simulink model "lab1_state_feedback_windup"  (R2024b)
settings: Solver=ode45  StartTime=0.0  StopTime=sIn.simulation_time
undefined symbols (not defined in the file or in its folder): degs2rpm, drv, feedback, filt, gbox, mld, mot, rads2rpm, rpm2rads, sens
libraries: simulink_extras x2, simulink x1
settings Model: Creator=bmm1  LastModifiedBy=pries
settings DataIOCC: ReturnWorkspaceOutputs=off
settings RTWCC: GPUComputeCapability=3.5

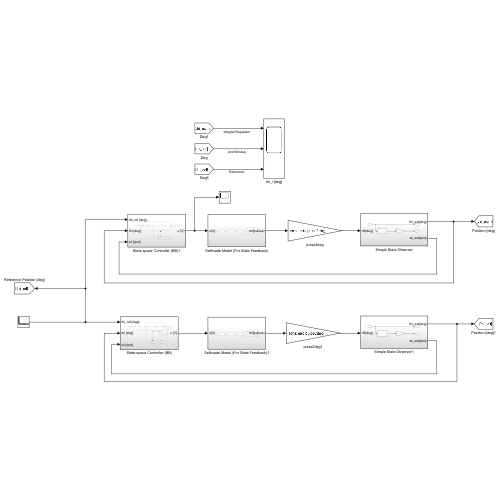
[thumbnail: Simulink's stored preview of the top-level diagram]
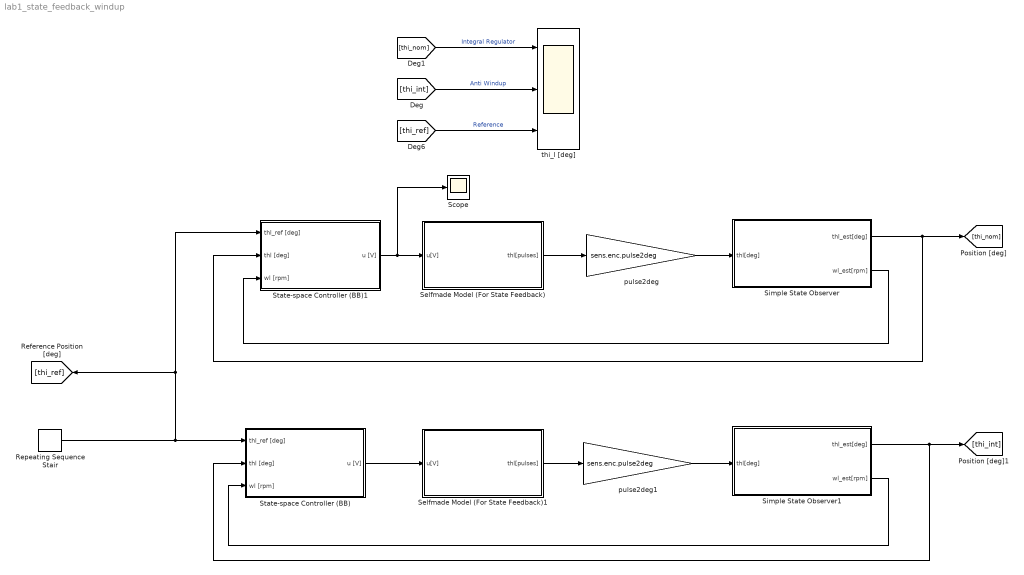
== system lab1_state_feedback_windup ==
  Repeating Sequence Stair : simulink/Sources/Repeating Sequence Stair  OutValues=sIn.position  tsamp=sIn.sample_time  OutMin=[]  OutMax=[]  OutDataTypeStr=double  OutputDataTypeScalingMode=double  OutDataType=fixdt(0,8)  ConRadixGroup=Best Precision: Vector-wise  OutScaling=2^-12
  Scope : Scope
  Selfmade Model (For State Feedback) : Subsystem
  Selfmade Model (For State Feedback)1 : Subsystem
  Simple State Observer : Subsystem
  Simple State Observer1 : Subsystem
  State-space Controller (BB) : Subsystem
  State-space Controller (BB)1 : Subsystem
  pulse2deg : Gain  Gain=sens.enc.pulse2deg
  pulse2deg1 : Gain  Gain=sens.enc.pulse2deg
  thi_l [deg] : Scope  NumInputPorts=3
  wires:
  Selfmade Model (For State Feedback)/1(thl[pulses]) -> pulse2deg/1
  Simple State Observer/1(thl_est[deg]) -> State-space Controller (BB)1/2(thl [deg]), [thi_nom]
  Simple State Observer/2(wl_est[rpm]) -> State-space Controller (BB)1/3(wl [rpm])
  State-space Controller (BB)1/1(u [V]) -> Scope/1, Selfmade Model (For State Feedback)/1(u[V])
  Repeating Sequence Stair/1 -> State-space Controller (BB)1/1(thl_ref [deg]), [thi_ref], State-space Controller (BB)/1(thl_ref [deg])
  State-space Controller (BB)/1(u [V]) -> Selfmade Model (For State Feedback)1/1(u[V])
  Selfmade Model (For State Feedback)1/1(thl[pulses]) -> pulse2deg1/1
  Simple State Observer1/1(thl_est[deg]) -> [thi_int], State-space Controller (BB)/2(thl [deg])
  Simple State Observer1/2(wl_est[rpm]) -> State-space Controller (BB)/3(wl [rpm])
  [thi_int] -> thi_l [deg]/2  "Anti Windup"
  [thi_nom] -> thi_l [deg]/1  "Integral Regulator"
  [thi_ref] -> thi_l [deg]/3  "Reference"
  pulse2deg1/1 -> Simple State Observer1/1(thl[deg])
  pulse2deg/1 -> Simple State Observer/1(thl[deg])

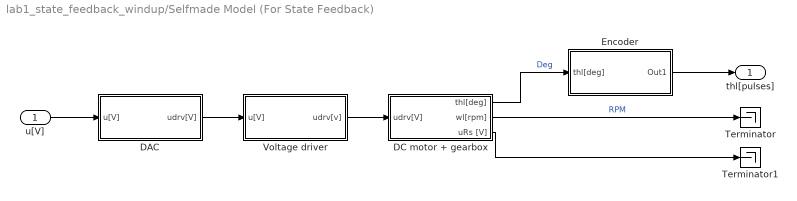
== system lab1_state_feedback_windup/Selfmade Model (For State Feedback) ==
  u[V] : Inport
  DAC : Subsystem
  DC motor + gearbox : Subsystem
  Encoder : Subsystem
  Terminator : Terminator
  Terminator1 : Terminator
  Voltage driver : Subsystem
  thl[pulses] : Outport
  wires:
  DC motor + gearbox/1(thl[deg]) -> Encoder/1(thl[deg])  "Deg"
  u[V]/1 -> DAC/1(u[V])
  DC motor + gearbox/2(wl[rpm]) -> Terminator/1  "RPM"
  DAC/1(udrv[V]) -> Voltage driver/1(u[V])
  Voltage driver/1(udrv[v]) -> DC motor + gearbox/1(udrv[V])
  Encoder/1(Out1) -> thl[pulses]/1
  DC motor + gearbox/3(uRs [V]) -> Terminator1/1

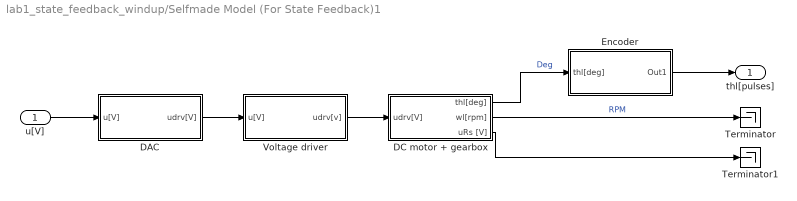
== system lab1_state_feedback_windup/Selfmade Model (For State Feedback)1 ==
  u[V] : Inport
  DAC : Subsystem
  DC motor + gearbox : Subsystem
  Encoder : Subsystem
  Terminator : Terminator
  Terminator1 : Terminator
  Voltage driver : Subsystem
  thl[pulses] : Outport
  wires:
  DC motor + gearbox/1(thl[deg]) -> Encoder/1(thl[deg])  "Deg"
  u[V]/1 -> DAC/1(u[V])
  DC motor + gearbox/2(wl[rpm]) -> Terminator/1  "RPM"
  DAC/1(udrv[V]) -> Voltage driver/1(u[V])
  Voltage driver/1(udrv[v]) -> DC motor + gearbox/1(udrv[V])
  Encoder/1(Out1) -> thl[pulses]/1
  DC motor + gearbox/3(uRs [V]) -> Terminator1/1

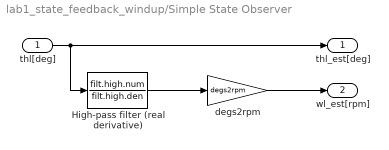
== system lab1_state_feedback_windup/Simple State Observer ==
  thl[deg] : Inport
  High-pass filter (real derivative) : TransferFcn  Numerator=filt.high.num  Denominator=filt.high.den
  degs2rpm : Gain  Gain=degs2rpm
  thl_est[deg] : Outport
  wl_est[rpm] : Outport  Port=2
  wires:
  thl[deg]/1 -> High-pass filter (real derivative)/1, thl_est[deg]/1
  High-pass filter (real derivative)/1 -> degs2rpm/1
  degs2rpm/1 -> wl_est[rpm]/1

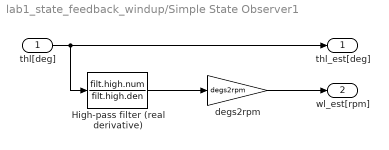
== system lab1_state_feedback_windup/Simple State Observer1 ==
  thl[deg] : Inport
  High-pass filter (real derivative) : TransferFcn  Numerator=filt.high.num  Denominator=filt.high.den
  degs2rpm : Gain  Gain=degs2rpm
  thl_est[deg] : Outport
  wl_est[rpm] : Outport  Port=2
  wires:
  thl[deg]/1 -> High-pass filter (real derivative)/1, thl_est[deg]/1
  High-pass filter (real derivative)/1 -> degs2rpm/1
  degs2rpm/1 -> wl_est[rpm]/1

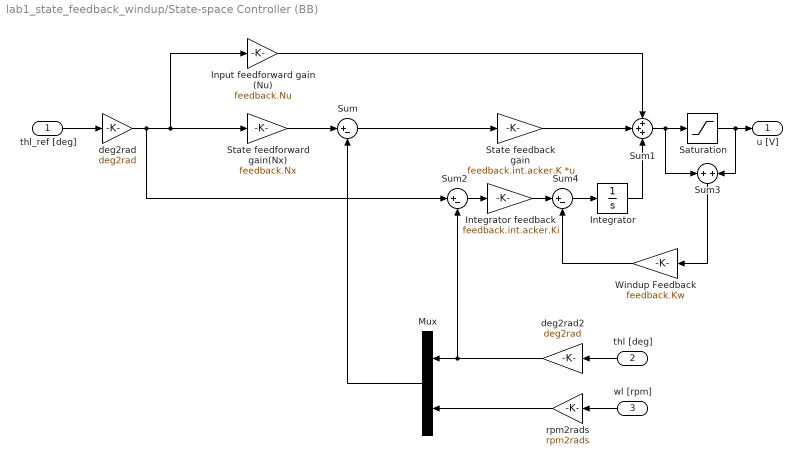
== system lab1_state_feedback_windup/State-space Controller (BB) ==
  thl_ref [deg] : Inport
  thl [deg] : Inport  Port=2
  wl [rpm] : Inport  Port=3
  Input feedforward gain (Nu) : Gain  Gain=feedback.Nu
  Integrator : Integrator
  Integrator feedback : Gain  Gain=feedback.int.acker.Ki
  Mux : Mux  Inputs=2
  Saturation : Saturate  UpperLimit=10  LowerLimit=-10
  State feedback gain : Gain  Gain=feedback.int.acker.K  Multiplication=Matrix(K*u)
  State feedforward gain(Nx) : Gain  Gain=feedback.Nx
  Sum : Sum  Inputs=|+-
  Sum1 : Sum  Inputs=+++
  Sum2 : Sum  Inputs=|+-
  Sum3 : Sum  Inputs=+|+
  Sum4 : Sum  Inputs=|+-
  Windup Feedback : Gain  Gain=feedback.Kw
  deg2rad : Gain  Gain=deg2rad
  deg2rad2 : Gain  Gain=deg2rad
  rpm2rads : Gain  Gain=rpm2rads
  u [V] : Outport
  wires:
  thl_ref [deg]/1 -> deg2rad/1
  deg2rad/1 -> Sum2/1, Input feedforward gain (Nu)/1, State feedforward gain(Nx)/1
  State feedforward gain(Nx)/1 -> Sum/1
  Sum/1 -> State feedback gain/1
  State feedback gain/1 -> Sum1/2
  Input feedforward gain (Nu)/1 -> Sum1/1
  Sum1/1 -> Sum3/1, Saturation/1
  Saturation/1 -> Sum3/2, u [V]/1
  thl [deg]/1 -> deg2rad2/1
  wl [rpm]/1 -> rpm2rads/1
  deg2rad2/1 -> Mux/1, Sum2/2
  rpm2rads/1 -> Mux/2
  Mux/1 -> Sum/2
  Sum2/1 -> Integrator feedback/1
  Integrator/1 -> Sum1/3
  Sum3/1 -> Windup Feedback/1
  Integrator feedback/1 -> Sum4/1
  Sum4/1 -> Integrator/1
  Windup Feedback/1 -> Sum4/2

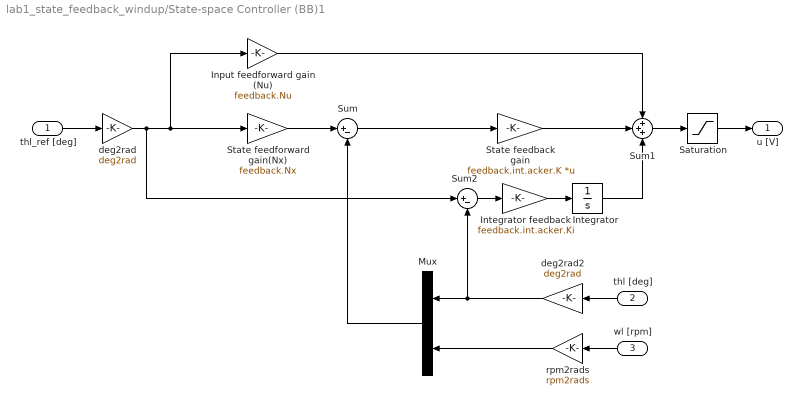
== system lab1_state_feedback_windup/State-space Controller (BB)1 ==
  thl_ref [deg] : Inport
  thl [deg] : Inport  Port=2
  wl [rpm] : Inport  Port=3
  Input feedforward gain (Nu) : Gain  Gain=feedback.Nu
  Integrator : Integrator
  Integrator feedback : Gain  Gain=feedback.int.acker.Ki
  Mux : Mux  Inputs=2
  Saturation : Saturate  UpperLimit=10  LowerLimit=-10
  State feedback gain : Gain  Gain=feedback.int.acker.K  Multiplication=Matrix(K*u)
  State feedforward gain(Nx) : Gain  Gain=feedback.Nx
  Sum : Sum  Inputs=|+-
  Sum1 : Sum  Inputs=+++
  Sum2 : Sum  Inputs=|+-
  deg2rad : Gain  Gain=deg2rad
  deg2rad2 : Gain  Gain=deg2rad
  rpm2rads : Gain  Gain=rpm2rads
  u [V] : Outport
  wires:
  thl_ref [deg]/1 -> deg2rad/1
  deg2rad/1 -> Sum2/1, Input feedforward gain (Nu)/1, State feedforward gain(Nx)/1
  State feedforward gain(Nx)/1 -> Sum/1
  Sum/1 -> State feedback gain/1
  State feedback gain/1 -> Sum1/2
  Input feedforward gain (Nu)/1 -> Sum1/1
  Sum1/1 -> Saturation/1
  Saturation/1 -> u [V]/1
  thl [deg]/1 -> deg2rad2/1
  wl [rpm]/1 -> rpm2rads/1
  deg2rad2/1 -> Sum2/2, Mux/1
  rpm2rads/1 -> Mux/2
  Mux/1 -> Sum/2
  Integrator feedback/1 -> Integrator/1
  Sum2/1 -> Integrator feedback/1
  Integrator/1 -> Sum1/3

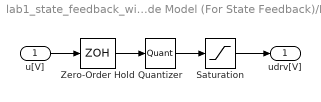
== system lab1_state_feedback_windup/Selfmade Model (For State Feedback)/DAC ==
  u[V] : Inport
  Quantizer : Quantizer  QuantizationInterval=daq.dac.q
  Saturation : Saturate  UpperLimit=10  LowerLimit=-10
  Zero-Order Hold : ZeroOrderHold  SampleTime=1e-3
  udrv[V] : Outport
  wires:
  Zero-Order Hold/1 -> Quantizer/1
  u[V]/1 -> Zero-Order Hold/1
  Quantizer/1 -> Saturation/1
  Saturation/1 -> udrv[V]/1

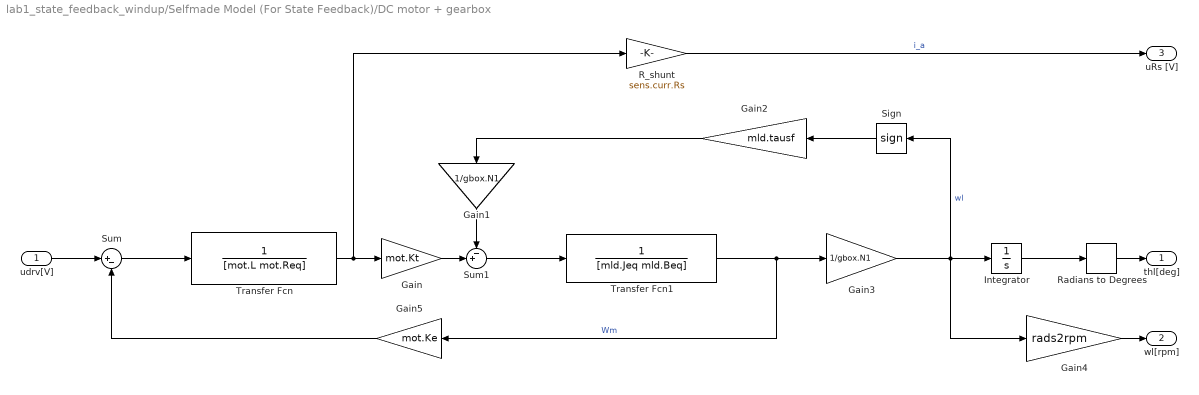
== system lab1_state_feedback_windup/Selfmade Model (For State Feedback)/DC motor + gearbox ==
  udrv[V] : Inport
  Gain : Gain  Gain=mot.Kt
  Gain1 : Gain  Gain=1/gbox.N1
  Gain2 : Gain  Gain=mld.tausf
  Gain3 : Gain  Gain=1/gbox.N1
  Gain4 : Gain  Gain=rads2rpm
  Gain5 : Gain  Gain=mot.Ke
  Integrator : Integrator
  R_shunt : Gain  Gain=sens.curr.Rs
  Radians to Degrees : simulink_extras/Transformations/Radians to Degrees
  Sign : Signum  ZeroCross=off
  Sum : Sum  Inputs=|+-
  Sum1 : Sum  Inputs=-+|
  Transfer Fcn : TransferFcn  Denominator=[mot.L mot.Req]
  Transfer Fcn1 : TransferFcn  Denominator=[mld.Jeq mld.Beq]
  thl[deg] : Outport
  wl[rpm] : Outport  Port=2
  uRs [V] : Outport  Port=3
  wires:
  udrv[V]/1 -> Sum/1
  Sum/1 -> Transfer Fcn/1
  Transfer Fcn/1 -> R_shunt/1, Gain/1
  Gain1/1 -> Sum1/1
  Gain2/1 -> Gain1/1
  Sign/1 -> Gain2/1
  Transfer Fcn1/1 -> Gain5/1, Gain3/1  "Wm"
  Gain3/1 -> Gain4/1, Sign/1, Integrator/1  "wl"
  Integrator/1 -> Radians to Degrees/1
  Radians to Degrees/1 -> thl[deg]/1
  Gain4/1 -> wl[rpm]/1
  Sum1/1 -> Transfer Fcn1/1
  Gain/1 -> Sum1/2
  Gain5/1 -> Sum/2
  R_shunt/1 -> uRs [V]/1  "i_a"

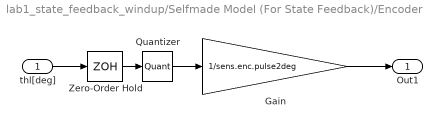
== system lab1_state_feedback_windup/Selfmade Model (For State Feedback)/Encoder ==
  thl[deg] : Inport
  Gain : Gain  Gain=1/sens.enc.pulse2deg
  Quantizer : Quantizer  QuantizationInterval=sens.enc.pulse2deg
  Zero-Order Hold : ZeroOrderHold  SampleTime=1e-3
  Out1 : Outport
  wires:
  thl[deg]/1 -> Zero-Order Hold/1
  Gain/1 -> Out1/1
  Quantizer/1 -> Gain/1
  Zero-Order Hold/1 -> Quantizer/1

== system lab1_state_feedback_windup/Selfmade Model (For State Feedback)/Voltage driver ==
  u[V] : Inport
  Saturation : Saturate  UpperLimit=12  LowerLimit=-12
  Transfer Fcn : TransferFcn  Numerator=[drv.dcgain]  Denominator=[drv.Tc 1]
  udrv[v] : Outport
  wires:
  u[V]/1 -> Transfer Fcn/1
  Transfer Fcn/1 -> Saturation/1
  Saturation/1 -> udrv[v]/1

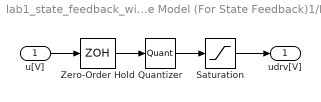
== system lab1_state_feedback_windup/Selfmade Model (For State Feedback)1/DAC ==
  u[V] : Inport
  Quantizer : Quantizer  QuantizationInterval=daq.dac.q
  Saturation : Saturate  UpperLimit=10  LowerLimit=-10
  Zero-Order Hold : ZeroOrderHold  SampleTime=1e-3
  udrv[V] : Outport
  wires:
  Zero-Order Hold/1 -> Quantizer/1
  u[V]/1 -> Zero-Order Hold/1
  Quantizer/1 -> Saturation/1
  Saturation/1 -> udrv[V]/1

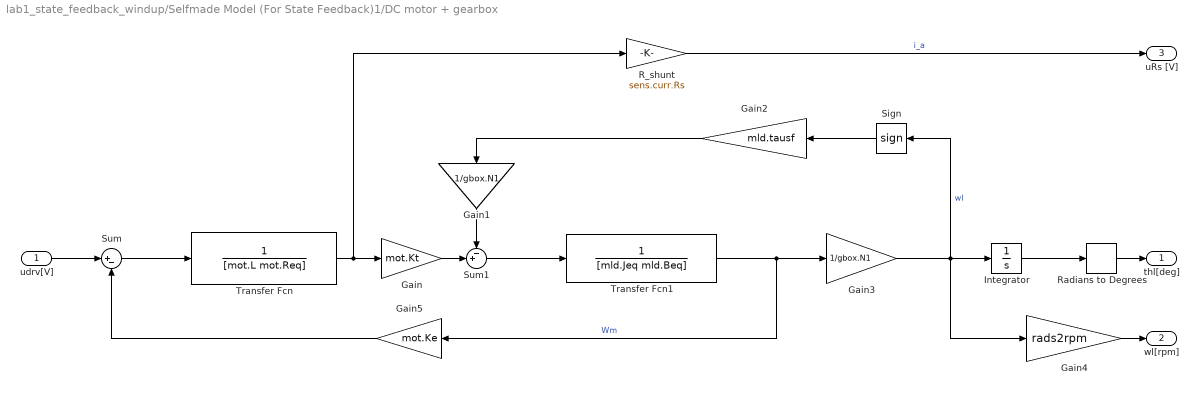
== system lab1_state_feedback_windup/Selfmade Model (For State Feedback)1/DC motor + gearbox ==
  udrv[V] : Inport
  Gain : Gain  Gain=mot.Kt
  Gain1 : Gain  Gain=1/gbox.N1
  Gain2 : Gain  Gain=mld.tausf
  Gain3 : Gain  Gain=1/gbox.N1
  Gain4 : Gain  Gain=rads2rpm
  Gain5 : Gain  Gain=mot.Ke
  Integrator : Integrator
  R_shunt : Gain  Gain=sens.curr.Rs
  Radians to Degrees : simulink_extras/Transformations/Radians to Degrees
  Sign : Signum  ZeroCross=off
  Sum : Sum  Inputs=|+-
  Sum1 : Sum  Inputs=-+|
  Transfer Fcn : TransferFcn  Denominator=[mot.L mot.Req]
  Transfer Fcn1 : TransferFcn  Denominator=[mld.Jeq mld.Beq]
  thl[deg] : Outport
  wl[rpm] : Outport  Port=2
  uRs [V] : Outport  Port=3
  wires:
  udrv[V]/1 -> Sum/1
  Sum/1 -> Transfer Fcn/1
  Transfer Fcn/1 -> R_shunt/1, Gain/1
  Gain1/1 -> Sum1/1
  Gain2/1 -> Gain1/1
  Sign/1 -> Gain2/1
  Transfer Fcn1/1 -> Gain5/1, Gain3/1  "Wm"
  Gain3/1 -> Gain4/1, Sign/1, Integrator/1  "wl"
  Integrator/1 -> Radians to Degrees/1
  Radians to Degrees/1 -> thl[deg]/1
  Gain4/1 -> wl[rpm]/1
  Sum1/1 -> Transfer Fcn1/1
  Gain/1 -> Sum1/2
  Gain5/1 -> Sum/2
  R_shunt/1 -> uRs [V]/1  "i_a"

== system lab1_state_feedback_windup/Selfmade Model (For State Feedback)1/Encoder ==
  thl[deg] : Inport
  Gain : Gain  Gain=1/sens.enc.pulse2deg
  Quantizer : Quantizer  QuantizationInterval=sens.enc.pulse2deg
  Zero-Order Hold : ZeroOrderHold  SampleTime=1e-3
  Out1 : Outport
  wires:
  thl[deg]/1 -> Zero-Order Hold/1
  Gain/1 -> Out1/1
  Quantizer/1 -> Gain/1
  Zero-Order Hold/1 -> Quantizer/1

== system lab1_state_feedback_windup/Selfmade Model (For State Feedback)1/Voltage driver ==
  u[V] : Inport
  Saturation : Saturate  UpperLimit=12  LowerLimit=-12
  Transfer Fcn : TransferFcn  Numerator=[drv.dcgain]  Denominator=[drv.Tc 1]
  udrv[v] : Outport
  wires:
  u[V]/1 -> Transfer Fcn/1
  Transfer Fcn/1 -> Saturation/1
  Saturation/1 -> udrv[v]/1
